simulink model "control"  (R2020b)
settings: Solver=VariableStepAuto  StartTime=0.0  StopTime=10.0  RelTol=1e-3
undefined symbols (not defined in the file or in its folder): DiscIntNeverNeededParam, dt_planner
settings Model: Creator=VVM  LastModifiedBy=VVM

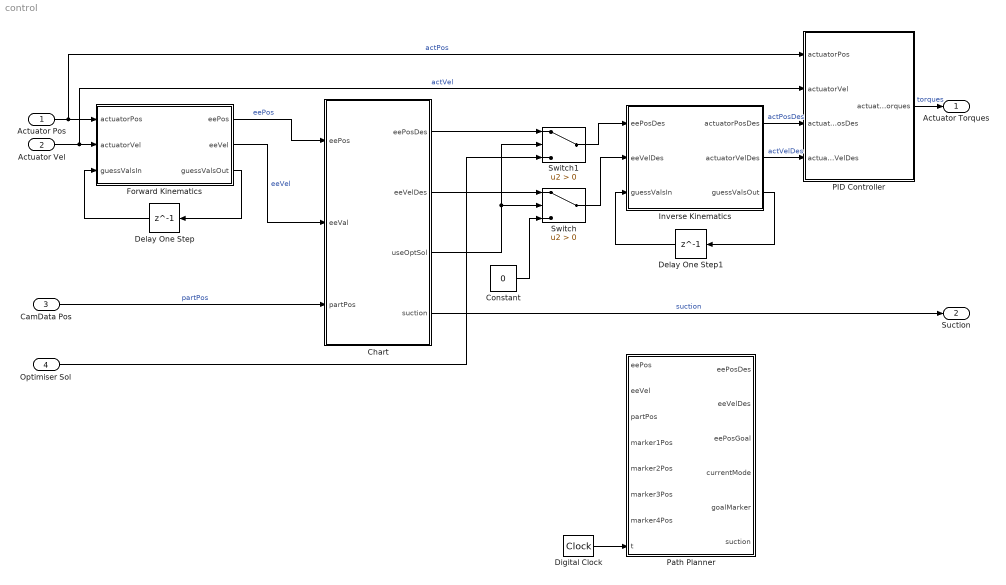
== system control ==
  Actuator Pos : Inport
  Actuator Vel : Inport  Port=2
  CamData Pos : Inport  Port=3
  Optimiser Sol : Inport  Port=4
  Chart : Stateflow chart  TreatAsAtomicUnit=on
  Constant : Constant  Value=0
  Delay One Step : Delay  DelayLength=1
  Delay One Step1 : Delay  DelayLength=1
  Digital Clock : DigitalClock  SampleTime=dt_planner
  Forward Kinematics : MATLAB Function  TreatAsAtomicUnit=on
  Inverse Kinematics : MATLAB Function  TreatAsAtomicUnit=on
  PID Controller : Subsystem  TreatAsAtomicUnit=on  mask(PID Controller){P=0.5, I=6, D=0.15}
  Path Planner : MATLAB Function  TreatAsAtomicUnit=on
  Switch : Switch  Criteria=u2 > Threshold
  Switch1 : Switch  Criteria=u2 > Threshold
  Actuator Torques : Outport
  Suction : Outport  Port=2
  wires:
  PID Controller/1(actuatorTorques) -> Actuator Torques/1  "torques"
  Forward Kinematics/3(guessValsOut) -> Delay One Step/1
  Inverse Kinematics/2(actuatorVelDes) -> PID Controller/4(actuatorVelDes)  "actVelDes"
  Actuator Vel/1 -> Forward Kinematics/2(actuatorVel), PID Controller/2(actuatorVel)  "actVel"
  Forward Kinematics/2(eeVel) -> Chart/2(eeVal)  "eeVel"
  Forward Kinematics/1(eePos) -> Chart/1(eePos)  "eePos"
  Inverse Kinematics/1(actuatorPosDes) -> PID Controller/3(actuatorPosDes)  "actPosDes"
  Chart/4(suction) -> Suction/1  "suction"
  Delay One Step1/1 -> Inverse Kinematics/3(guessValsIn)
  Inverse Kinematics/3(guessValsOut) -> Delay One Step1/1
  CamData Pos/1 -> Chart/3(partPos)  "partPos"
  Delay One Step/1 -> Forward Kinematics/3(guessValsIn)
  Actuator Pos/1 -> Forward Kinematics/1(actuatorPos), PID Controller/1(actuatorPos)  "actPos"
  Chart/2(eeVelDes) -> Switch/1
  Switch/1 -> Inverse Kinematics/2(eeVelDes)
  Constant/1 -> Switch/3
  Chart/3(useOptSol) -> Switch1/2, Switch/2
  Switch1/1 -> Inverse Kinematics/1(eePosDes)
  Chart/1(eePosDes) -> Switch1/1
  Optimiser Sol/1 -> Switch1/3
  Digital Clock/1 -> Path Planner/8(t)

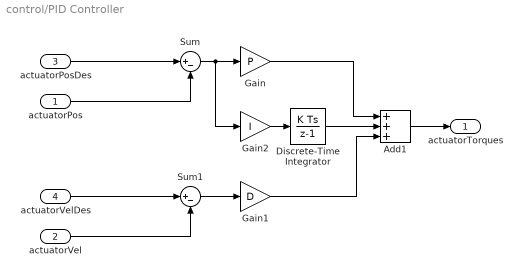
== system control/PID Controller ==
  actuatorPos : Inport
  actuatorVel : Inport  Port=2
  actuatorPosDes : Inport  Port=3
  actuatorVelDes : Inport  Port=4
  Add1 : Sum  Inputs=+++
  Discrete-Time Integrator : DiscreteIntegrator  gainval=1  SampleTime=-1  ICPrevOutput=DiscIntNeverNeededParam  ICPrevScaledInput=DiscIntNeverNeededParam
  Gain : Gain  Gain=P
  Gain1 : Gain  Gain=D
  Gain2 : Gain  Gain=I
  Sum : Sum  Inputs=|+-
  Sum1 : Sum  Inputs=|+-
  actuatorTorques : Outport
  wires:
  actuatorPosDes/1 -> Sum/1
  actuatorPos/1 -> Sum/2
  actuatorVel/1 -> Sum1/2
  Sum/1 -> Gain2/1, Gain/1
  Sum1/1 -> Gain1/1
  Gain/1 -> Add1/1
  Gain1/1 -> Add1/3
  Discrete-Time Integrator/1 -> Add1/2
  Gain2/1 -> Discrete-Time Integrator/1
  Add1/1 -> actuatorTorques/1
  actuatorVelDes/1 -> Sum1/1

== matlab function control/Path Planner ==
  data: eePos input size=3; eePosDes output size=3; eeVel input size=3; partPos input size=3; marker1Pos input size=3; marker2Pos input size=3; marker3Pos input size=3; marker4Pos input size=3; t input size=1; eeVelDes output size=3; eePosGoal output; currentMode output size=1; goalMarker output size=1; suction output size=1
function [eePosDes, eeVelDes, eePosGoal, currentMode, goalMarker, suction] = Planner(eePos, eeVel, partPos, marker1Pos, marker2Pos, marker3Pos, marker4Pos, t)
% Top-level planner.  The end effector goal and suction state depend on
% the current mode: 
%
% mode 0: go to home/initial position (suction off)
% mode 1: go to part (suction off)
% mode 2: move part to goal position (suction on)
%
% When a mode is first entered, a 3rd order polynomial curve c(s) is
% computed corresponding to the desired path (in xyz camera coordinates) of
% the end effector from its current position to the goal position for that
% mode. Additionally, a 5th order polynomial s(t) is computed which serves
% as the time-scaling along the path.  The time-scaling is computed such
% that the initial and final velocities and accelerations along the path
% are zero. This results in a desired trajectory c(s(t)) = c(t).  For a
% given time, this function returns the corresponding position (c(t) =
% eePosDes) and velocity (c'(t) = eeVelDes) of the trajectory.

% Copyright 2020 The MathWorks, Inc.

persistent mode homePos pickAndDropZGoal ...
    marker1PosGoal marker2PosGoal marker3PosGoal marker4PosGoal ...
    nextMarker stayHome

if isempty(mode)
    mode = 0;
    pickAndDropZGoal = partPos(3) - 0.001;
    marker1PosGoal = [marker1Pos(1:2); pickAndDropZGoal];
    marker2PosGoal = [marker2Pos(1:2); pickAndDropZGoal];
    marker3PosGoal = [marker3Pos(1:2); pickAndDropZGoal];
    marker4PosGoal = [marker4Pos(1:2); pickAndDropZGoal];
    homePos = eePos;
    nextMarker = 0;
    stayHome = false;
end

switch mode
    case 0
        % Go to home position
        suction = 0;
        eePosGoal = homePos;
        startVertical = true;
        endVertical = false;
        [eePosDes, eeVelDes, done] = gotoPosition(eePosGoal, eePos, eeVel, t, startVertical, endVertical);
        if done
            if ~stayHome
                mode = 1;
            end
        end
        
    case 1
        % Move to just above part and hover (end of path is vertical)
        eePosGoal = [partPos(1:2); pickAndDropZGoal];
        suction = 0;
        startVertical = false;
        endVertical = true;
        [eePosDes, eeVelDes, done] = gotoPosition(eePosGoal, eePos, eeVel, t, startVertical, endVertical);
        if done
            nextMarker = 1;
            mode = 2;
        end
        
    case 2
        % Grasp part and move it to the next marker (beginning and end of
        % path are vertical)
        switch nextMarker
            case 1
                eePosGoal = marker1PosGoal;
            case 2
                eePosGoal = marker2PosGoal;
            case 3
                eePosGoal = marker3PosGoal;
            case 4
                eePosGoal = marker4PosGoal;
            otherwise
                error('invalid nextMarker')
        end
        suction = 1;
        startVertical = true;
        endVertical = true;
        [eePosDes, eeVelDes, done] = gotoPosition(eePosGoal, eePos, eeVel, t, startVertical, endVertical);
        if done
            nextMarker = nextMarker + 1;
            if nextMarker == 5
                nextMarker = 1;
                stayHome = true;
            end
            if nextMarker == 2 && stayHome
                nextMarker = 0;
                mode = 0;
            end
        end
        
    otherwise
        error('invalid mode')
end

currentMode = mode;
goalMarker = nextMarker;
end


function p = getPoly5(t0,tf,x0,v0,a0,xf,vf,af)
% Compute the 5th order polynomial 
% 
% poly(t) = a*t^5 + b*t^4 + c*t^3 + d*t^2 + e*t + f
%
% such that
%
% p(t0) = x0; p(tf) = xf
% p'(t0) = v0; p'(tf) = vf
% p''(to) = a0; p''(tf) = af
%
% Returns the coeffecient vector p = [a b c d e f]

A = [t0^5    t0^4    t0^3   t0^2 t0 1;
     5*t0^4  4*t0^3  3*t0^2 2*t0 1  0;
     20*t0^3 12*t0^2 6*t0   2    0  0;
     tf^5    tf^4    tf^3   tf^2 tf 1;
     5*tf^4  4*tf^3  3*tf^2 2*tf 1  0;
     20*tf^3 12*tf^2 6*tf   2    0  0];
b = [x0 v0 a0 xf vf af]';
p = A\b;
end

function p = getPoly3(t0,tf,x0,v0,xf,vf)
% Compute the 3rd order polynomial 
% 
% poly(t) = a*t^3 + b*t^2 + c*t + d
%
% such that
%
% p(t0) = x0; p(tf) = xf
% p'(t0) = v0; p'(tf) = vf
%
% Returns the coeffecient vector p = [a b c d]

A = [t0^3   t0^2 t0 1;
     3*t0^2 2*t0 1  0;
     tf^3   tf^2 tf 1;
     3*tf^2 2*tf 1  0];
b = [x0 v0 xf vf]';
p = A\b;
end

function [eePosDes, eeVelDes, atGoal] = gotoGoal(...
    plan, ...
    t, timeToGoal, ...
    eePos, eeVel, ...
    eePosGoal, startDirectionGoal, endDirectionGoal)
% Return desired position and and velocity at current time along the
% trajectory to a goal position.  The trajectory is only computed is 'plan'
% is true.  The trajectory is determined by the desired time to reach the
% goal (timeToGoal), the desired goal position (eePosGoal), and the
% starting and ending directions (startDirectionGoal and endDirectionGoal)
% of the curve to the goal in xyz camera coordinates.  It always assumed
% that the initial and final velocities and accelerations along the
% trajectory are zero.  Thus, the goal velocity is always zero.  If the
% current position and velocity are sufficiently close to the goal position
% and velocity, 'atGoal' is true.

persistent cpoly cdpoly spoly sdpoly t0 tf ...
    maxErrPos maxErrVel

if isempty(tf)
    cpoly = zeros(3,4);
    cdpoly = zeros(3,3);
    spoly = zeros(1,6);
    sdpoly = zeros(1,5);
    
    t0 = t;
    tf = t;
    
    maxErrPos = 0.002;
    maxErrVel = 0.01;
end

errPos = eePosGoal - eePos;
errVel = -eeVel;
errPosNorm = norm(errPos);
errVelNorm = norm(errVel);

if plan
    t0 = t;
    tf = t0 + timeToGoal;
    [cpoly, cdpoly, spoly, sdpoly] = getTrajectory(...
        t0, tf, eePos, eePosGoal, startDirectionGoal, endDirectionGoal);
end

t = min(t,tf); %if t > tf, we just want to keep aiming for end of trajectory
s = polyval(spoly,t);
eePosDes = [polyval(cpoly(1,:),s);polyval(cpoly(2,:),s);polyval(cpoly(3,:),s)];
eeVelDes = [polyval(cdpoly(1,:),s);polyval(cdpoly(2,:),s);polyval(cdpoly(3,:),s)]*polyval(sdpoly,t);
atGoal = errPosNorm < maxErrPos && errVelNorm < maxErrVel;
end

function [cpoly, cdpoly, spoly, sdpoly] = getTrajectory(...
    t0, tf, eePos, eePosGoal, startDirectionGoal, endDirectionGoal)
% Return polynomials needed to compute a time-scaled trajectory
% from eePos to eePosGoal such that initial and final velocities
% and accelerations are zero.  The path of the trajectory in xyz space has
% an initial tangent equal to startDirectionGoal and an ending tangent of
% endDirectionGoal.
%
% Let c(s) = [x(s);y(s);z(s)] with s = [0 1] be a curve in xyz space from
% eePos to eePosGoal.  We assume each element is a 3rd order
% polymonial and compute the corresponding 3-by-4 coefficient matrix,
% cpoly:
%
%         [a1*s^3 + b1*s^2 + c1*s + d1]           [s^3]
%  c(s) = [a2*s^3 + b2*s^2 + c2*s + d2] = cpoly * [s^2]
%         [a3*s^3 + b3*s^2 + c3*s + d3]           [s  ]
%                                                 [1  ]
%
% The 12 coefficeints in cpoly are uniquely determined by the following
% boundary conditions:
%
% c(0) = eePos
% c(1) = eePosGoal
% c'(0) = startDirectionGoal
% c'(1) = endDirectionGoal
%
% cdpoly is a 3-by-3 matrix of polynomial coefficents of the derivatives of
% each row of cpoly:
%
%          [3*a1 2*b1 c1]
% cdpoly = [3*a2 2*b2 c2]
%          [3*a3 2*b3 c3]
%
% The curve c(s) is then time-scaled to ensure that the initial and final
% speeds and accelerations along the curve are zero.  The time scaling
% s(t) is a 5th order polynomial
%
%  s(t) = A*s^5 + B*s^4 + C*s^3 + D*s^2 + E*s + F
%
%       = spoly*[s^5 s^4 s^3 s^2 s 1]'
%
% spoly is a 1-by-6 vector of coefficents with values uniquely determined
% by the following boundary conditions:
%
% s(t0) = 0
% s(tf) = 1
% s'(t0) = 0
% s'(tf) = 0
% s''(t0) = 0
% s''(tf) = 0
%
% sdpoly is a 1-by-5 matrix of polynomial coefficents of the derivative of
% spoly:
%
% sdpoly = [5*A 4*B 3*C 2*D E]
%
% The final time-scaled trajectory corresponds to c(s(t))

s0 = 0;
sf = 1;
c0 = eePos;
cf = eePosGoal;
cd0 = startDirectionGoal;
cdf = endDirectionGoal;
cpoly = zeros(3,4);
cdpoly = zeros(3,3);
for i = 1:3
    cpoly(i,:) = getPoly3(s0,sf,c0(i),cd0(i),cf(i),cdf(i));
    % Need to be careful with polyder.  If the polynomial is equivalent
    % to just a constant (e.g., [0 0 0 1]), then polyder returns [0]
    % instead of [0 0 0].
    pd = polyder(cpoly(i,:));
    if length(pd) == 3
        cdpoly(i,:) = pd;
    else
        cdpoly(i,:) = [0 0 0];
    end
end

s0 = 0;
sf = 1;
sd0 = 0;
sdf = 0;
sdd0 = 0;
sddf = 0;
spoly = getPoly5(t0,tf,s0,sd0,sdd0,sf,sdf,sddf);
sdpoly = polyder(spoly);
end

function [eePosDes, eeVelDes, done] = gotoPosition(eePosGoal, eePos, eeVel, t, startVertical, endVertical)
% High-level function to go to a goal position.  Returns the desired
% position and and velocity at current time along the trajectory to a goal
% position. The time to goal along the trajectory is always set to 0.2
% seconds. startVertical and endVertical indicate whether the curve defined
% by the trajectory should begin and/or end vertically (i.e., the end
% effector should move straight up or down when starting or ending its
% motion).  It always assumed that the initial and final velocities and
% accelerations along the trajectory are zero.  Thus, the goal velocity is
% always zero. If the current position and velocity are sufficiently close
% to the goal position and velocity, 'done' is true.

persistent plan
if isempty(plan)
    plan = true;
end

if startVertical
    startDirectionGoal = [0;0;-0.2];
else
    startDirectionGoal = eeVel;
end
if endVertical
    endDirectionGoal = [0;0;0.2];
else
    endDirectionGoal = [0;0;0];
end
timeToGoal = 0.2;
[eePosDes, eeVelDes, atGoal] = gotoGoal(...
    plan, ...
    t, timeToGoal, ...
    eePos, eeVel, ...
    eePosGoal, startDirectionGoal, endDirectionGoal);
plan = atGoal;
done = atGoal;
end

== stateflow chart control/Chart ==
  data: eePos input; eeVal input; partPos input; eePosDes output; eeVelDes output; useOptSol output; suction output

== matlab function control/Forward Kinematics ==
  data: actuatorPos input size=3; eePos output size=3; actuatorVel input size=3; guessValsIn input size=3; eeVel output; guessValsOut output size=3
function [eePos, eeVel, guessValsOut] = FK(actuatorPos, actuatorVel, guessValsIn)
% Wrapper around sm_pick_and_place_fk.m, which creates a persistent
% KinematicsSolver object for the forwards kinematics problem and then
% solves it.

coder.extrinsic('sm_pick_and_place_robot_fk');
persistent init
if isempty(init)
    init = true;
    eePos = zeros(3,1);
    eeVel = zeros(3,1);
    guessValsOut = zeros(3,1);
    status = 1;
end
[eePos, eeVel, guessValsOut, status] = sm_pick_and_place_robot_fk(actuatorPos, actuatorVel, guessValsIn);
if status ~= 1
    error('fk solve failed')
end

== matlab function control/Inverse Kinematics ==
  data: eePosDes input size=3; actuatorPosDes output size=3; eeVelDes input size=3; guessValsIn input size=3; actuatorVelDes output size=3; guessValsOut output size=3
function [actuatorPosDes, actuatorVelDes, guessValsOut] = IK(eePosDes, eeVelDes, guessValsIn)
% Wrapper around sm_pick_and_place_ik.m, which creates a persistent
% KinematicsSolver object for the inverse kinematics problem and then
% solves it.

coder.extrinsic('sm_pick_and_place_robot_ik');
persistent init
if isempty(init)
    init = true;
    actuatorPosDes = zeros(3,1);
    actuatorVelDes = zeros(3,1);
    guessValsOut = zeros(3,1);
    status = 1;
end
[actuatorPosDes, actuatorVelDes, guessValsOut, status] = sm_pick_and_place_robot_ik(eePosDes, eeVelDes, guessValsIn);
if status ~= 1
    error('ik solve failed');
end
